simulink model "AA3"  (R2021a)
settings: Solver=VariableStepAuto  StartTime=0.0  StopTime=500  RelTol=1e-3
libraries: simulink x1
settings Model: Creator=jhaid  LastModifiedBy=jhaid

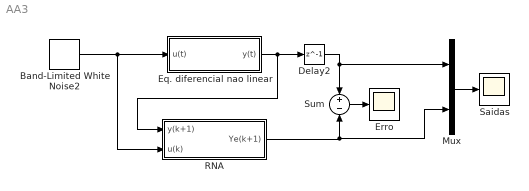
== system AA3 ==
  Band-Limited White Noise2 : simulink/Sources/Band-Limited White Noise  Cov=[10]  Ts=1  seed=[21]
  Delay2 : Delay  DelayLength=1
  Eq. diferencial nao linear : Subsystem
  Erro : Scope
  Mux : Mux  Inputs=2
  RNA : Subsystem  mask{Alfa=0.1, T=1, Wini=[ 1.544 -0.8868 0.04979 0.08669 0.1863 0.02026], Wnet=[ 1.544 -0.8868 0.04979 0.08669 0.1863 0.02026]}
      mask prompts: Alfa "LearningRate"; T "Treina/Opera(1/0)"; Wini "Pesos Iniciais"; Wnet "Pesos Treinados"
  Saidas : Scope
  Sum : Sum  Inputs=+|-
  wires:
  Sum/1 -> Erro/1
  Eq. diferencial nao linear/1(y(t)) -> Delay2/1, RNA/1(y(k+1))
  Delay2/1 -> Sum/1, Mux/1
  Mux/1 -> Saidas/1
  Band-Limited White Noise2/1 -> Eq. diferencial nao linear/1(u(t)), RNA/2(u(k))
  RNA/1(Ye(k+1)) -> Mux/2, Sum/2

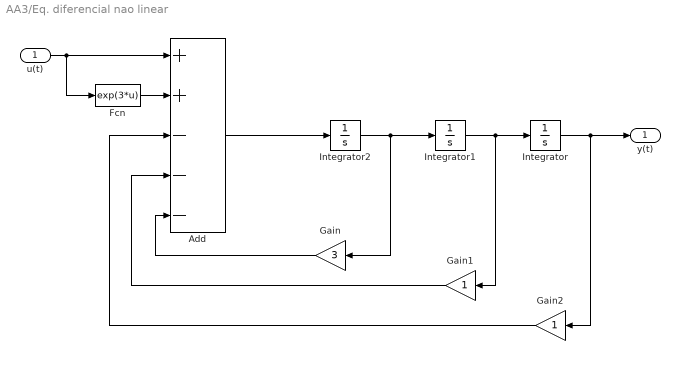
== system AA3/Eq. diferencial nao linear ==
  u(t) : Inport
  Add : Sum  Inputs=++---
  Fcn : Fcn  Expr=exp(3*u)
  Gain : Gain  Gain=3
  Gain1 : Gain
  Gain2 : Gain
  Integrator : Integrator
  Integrator1 : Integrator
  Integrator2 : Integrator
  y(t) : Outport
  wires:
  Add/1 -> Integrator2/1
  Integrator/1 -> y(t)/1, Gain2/1
  Integrator1/1 -> Integrator/1, Gain1/1
  Integrator2/1 -> Integrator1/1, Gain/1
  u(t)/1 -> Fcn/1, Add/1
  Gain/1 -> Add/5
  Gain1/1 -> Add/4
  Gain2/1 -> Add/3
  Fcn/1 -> Add/2

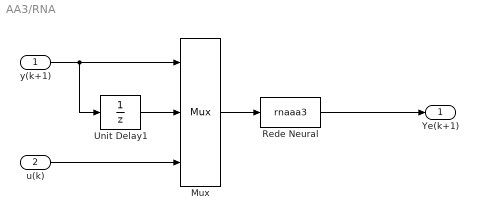
== system AA3/RNA ==
  y(k+1) : Inport
  u(k) : Inport  Port=2
  Mux : Mux  Inputs=3
  Rede Neural : S-Function  FunctionName=rnaaa3  SFunctionDeploymentMode=off  EnableBusSupport=off
  Unit Delay1 : UnitDelay  SampleTime=-1  HasFrameUpgradeWarning=on
  Ye(k+1) : Outport  VectorParamsAs1DForOutWhenUnconnected=off
  wires:
  y(k+1)/1 -> Mux/1, Unit Delay1/1
  u(k)/1 -> Mux/3
  Unit Delay1/1 -> Mux/2
  Mux/1 -> Rede Neural/1
  Rede Neural/1 -> Ye(k+1)/1
